simulink model "simulink_implementation"  (R2019b)
settings: Solver=FixedStepDiscrete  StartTime=0.0  StopTime=timetorun  RelTol=1e-3
undefined symbols (not defined in the file or in its folder): buffer_ratio, DiscIntNeverNeededParam, dsp_slices, sample_rate
libraries: simulink x3, hdlsllib x2, dspsrcs4 x1
settings Model: DataTypeOverride=Off  Creator=ian  LastModifiedBy=ian
settings DataIOCC: LimitDataPoints=on  SaveOutput=off  SaveTime=off
settings OptimizationCC: BlockReduction=off  ConditionallyExecuteInputs=off  DefaultParameterBehavior=Inlined  LifeSpan=inf
settings DebuggingCC: SignalRangeChecking=warning  AlgebraicLoopMsg=error  SingleTaskRateTransMsg=error  AllowSymbolicDim=off  StrictBusMsg=ErrorOnBusTreatedAsVector  SFUnexpectedBacktrackingDiag=warning  SFNoUnconditionalDefaultTransitionDiag=warning  SFExecutionAtInitializationDiag=none  ArithmeticOperatorsInVariantConditions=warning
settings HardwareCC: ProdBitPerPointer=32  ProdBitPerSizeT=32  ProdBitPerPtrDiffT=32  ProdLargestAtomicFloat=None  ProdIntDivRoundTo=Undefined  ProdEndianess=Unspecified  ProdWordSize=32  ProdHWDeviceType=ASIC/FPGA->ASIC/FPGA  TargetBitPerPointer=64  TargetBitPerSizeT=64  TargetBitPerPtrDiffT=64  TargetLongLongMode=on  TargetIntDivRoundTo=Zero  TargetEndianess=LittleEndian  TargetWordSize=64  TargetHWDeviceType=Custom Processor->MATLAB Host Computer  ProdEqTarget=off
settings SFSimCC: SimUseLocalCustomCode=off  CustomCodeUndefinedFunction=UseInterfaceOnly
settings RTWCC: RTWUseLocalCustomCode=off
settings CodeAppCC: StateflowObjectComments=on
settings GRTTargetCC: TargetLangStandard=C89/C90 (ANSI)  GeneratePreprocessorConditionals=Disable all
settings ConfigComp: CovScope=ReferencedModels  CovMetricSettings=dw  CovHtmlReporting=on  CovSaveCumulativeToWorkspaceVar=on  CovSaveSingleToWorkspaceVar=on  CovExternalEMLEnable=off  CovSFcnEnable=off

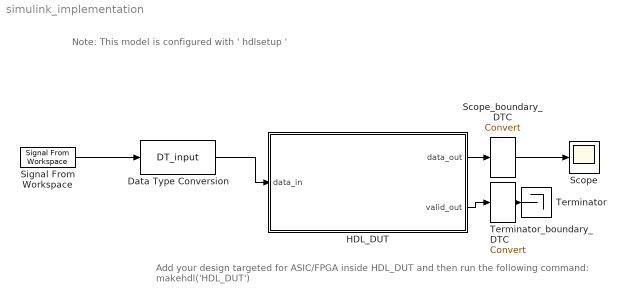
== system simulink_implementation ==
  note: Note: This model is configured with ' hdlsetup '
  note: Add your design targeted for ASIC/FPGA inside HDL_DUT and then run the following command:
      | makehdl('HDL_DUT')
  Data Type Conversion : DataTypeConversion  OutDataTypeStr=DT_input
  HDL_DUT : Subsystem
  Scope : Scope
  Scope_boundary_DTC : DataTypeConversion  SaturateOnIntegerOverflow=on  RndMeth=Zero
  Signal From Workspace : dspsrcs4/Signal From Workspace  X=v_in  Ts=sample_rate  nsamps=dsp_slices  OutputAfterFinalValue=Setting to zero  ignoreOrWarnInputAndFrameLengths=off  OutputFrames=off
  Terminator : Terminator
  Terminator_boundary_DTC : DataTypeConversion  SaturateOnIntegerOverflow=on  RndMeth=Zero
  wires:
  Signal From Workspace/1 -> Data Type Conversion/1
  Data Type Conversion/1 -> HDL_DUT/1(data_in)
  HDL_DUT/1(data_out) -> Scope_boundary_DTC/1
  Scope_boundary_DTC/1 -> Scope/1
  HDL_DUT/2(valid_out) -> Terminator_boundary_DTC/1
  Terminator_boundary_DTC/1 -> Terminator/1

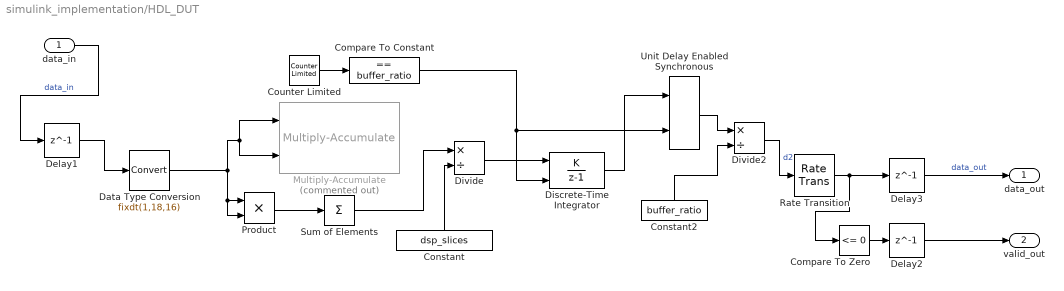
== system simulink_implementation/HDL_DUT ==
  data_in : Inport
  Compare To Constant : simulink/Logic and Bit Operations/Compare To Constant  relop===  const=buffer_ratio  OutDataTypeStr=boolean
  Compare To Zero : simulink/Logic and Bit Operations/Compare To Zero  relop=<=  OutDataTypeStr=boolean
  Constant : Constant  Value=dsp_slices  OutDataTypeStr=uint16  SampleTime=-1
  Constant2 : Constant  Value=buffer_ratio  OutDataTypeStr=uint16  SampleTime=-1
  Counter Limited : simulink/Sources/Counter Limited  uplimit=buffer_ratio  tsamp=-1
  Data Type Conversion : DataTypeConversion  OutDataTypeStr=fixdt(1,18,16)  RndMeth=Nearest
  Delay1 : Delay  DelayLength=1  InputProcessing=Columns as channels (frame based)
  Delay2 : Delay  DelayLength=1
  Delay3 : Delay  DelayLength=1
  Discrete-Time Integrator : DiscreteIntegrator  IntegratorMethod=Accumulation: Forward Euler  gainval=1  ExternalReset=falling  SampleTime=-1  LimitOutput=on  UpperSaturationLimit=1000  LowerSaturationLimit=0  ICPrevOutput=DiscIntNeverNeededParam  ICPrevScaledInput=DiscIntNeverNeededParam
  Divide : Product  Inputs=*/  SaturateOnIntegerOverflow=on  RndMeth=Zero
  Divide2 : Product  Inputs=*/  RndMeth=Simplest  SaturateOnIntegerOverflow=on
  Multiply-Accumulate : hdlsllib/HDL Operations/Multiply-Accumulate  Commented=on  opMode=Vector  initValueSetting=Dialog  initValue=0  initValueSetting2=Dialog  initValue2=0  initValueSetting3=Dialog  initValue3=0  num_samples=5  RndMeth=Nearest  RndMeth2=Floor  RndMeth3=Floor  OutDataTypeStr=MAC_out  datatype2=Inherit: Inherit via back propagation  datatype3=fixdt(1,16,0)  validOut=on  endInandOut=on  startOut=on  countOut=on  dim=-1  DoSatur=off  parallel=off
      settings: SourceProductName=Simulink  SourceProductBaseCode=SL
  Product : Product
  Rate Transition : RateTransition  OutPortSampleTimeOpt=Multiple of input port sample time  OutPortSampleTimeMultiple=buffer_ratio  OutPortSampleTime=average_duration
  Sum of Elements : Sum  Inputs=+
  Unit Delay Enabled Synchronous : hdlsllib/Discrete/Unit Delay Enabled Synchronous  InitialCondition=0.0  SampleTime=-1
      settings: SourceProductName=Simulink  SourceProductBaseCode=SL
  data_out : Outport  VectorParamsAs1DForOutWhenUnconnected=off
  valid_out : Outport  Port=2  VectorParamsAs1DForOutWhenUnconnected=off
  wires:
  data_in/1 -> Delay1/1  "data_in"
  Constant/1 -> Divide/2
  Delay1/1 -> Data Type Conversion/1
  Delay2/1 -> valid_out/1
  Counter Limited/1 -> Compare To Constant/1
  Unit Delay Enabled Synchronous/1 -> Divide2/1
  Divide2/1 -> Rate Transition/1  "d2"
  Constant2/1 -> Divide2/2
  Compare To Constant/1 -> Discrete-Time Integrator/2, Unit Delay Enabled Synchronous/2
  Rate Transition/1 -> Compare To Zero/1, Delay3/1
  Delay3/1 -> data_out/1  "data_out"
  Divide/1 -> Discrete-Time Integrator/1
  Discrete-Time Integrator/1 -> Unit Delay Enabled Synchronous/1
  Compare To Zero/1 -> Delay2/1
  Product/1 -> Sum of Elements/1
  Sum of Elements/1 -> Divide/1
  Data Type Conversion/1 -> Multiply-Accumulate/2, Multiply-Accumulate/1, Product/1, Product/2
